simulink model "Custom_Inverter_Working_1 1"  (R2024a)
settings: Solver=FixedStepAuto  StartTime=0.0  StopTime=40  FixedStep=1e-5  MaxStep=1e-4  RelTol=1e-3
values from neighbouring files (symbols this model uses):
  A_f = 1.24    [Inverter_Working 1.m]
  C_d = 0.7041    [Inverter_Working 1.m]
  C_rr = 0.02    [Inverter_Working 1.m]
  g = 9.8    [Inverter_Working 1.m]
  J = mrot*r^2/k^2 + 0.0045    (= 0.8303048)    [Inverter_Working 1.m]
  k = 1    [Inverter_Working 1.m]
  lambda = 0.0375    [Inverter_Working 1.m]
  Ld = 0.1e-3    (= 0.0001)    [Inverter_Working 1.m]
  Lq = Ld    (= 0.0001)    [Inverter_Working 1.m]
  m = 371    [Inverter_Working 1.m]
  ppair = 1    [Inverter_Working 1.m]
  r = 0.4064/2    (= 0.2032)    [Inverter_Working 1.m]
  rho = 1.2    [Inverter_Working 1.m]
  Rs = 1.3e-3    (= 0.0013)    [Inverter_Working 1.m]
  V_bat = 24 * 3.6    (= 86.4)    [Inverter_Working 1.m]
undefined symbols (not defined in the file or in its folder): Down, Up
libraries: nesl_utility x12, fl_lib x6, ee_lib x5, slpidlib x3, simulink x2, spsabctodq0Lib x2, spsdq0toabcLib x2, eePwmGenerator x1
settings Model: Creator=cviana  LastModifiedBy=didad
settings RTWCC: GPUComputeCapability=3.5

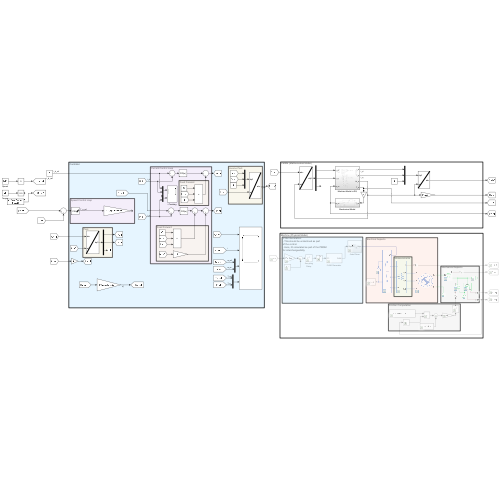
[thumbnail: Simulink's stored preview of the top-level diagram]
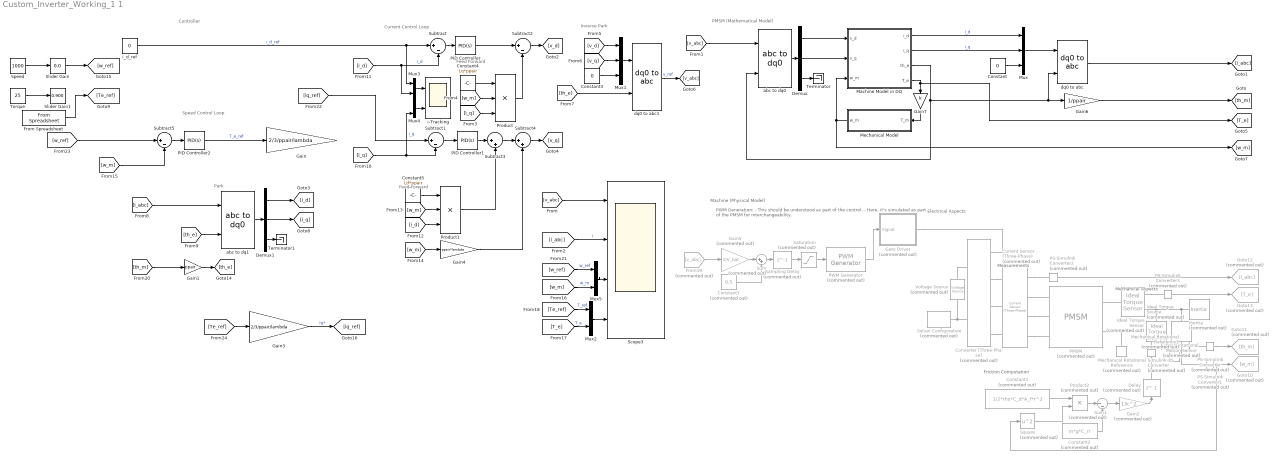
== system Custom_Inverter_Working_1 1 ==
  note: Friction Computation
  note: Machine (Physical Model)
  note: Feed Forward
  note: Feed Forward
  note: Current Control Loop
  note: Speed Control Loop
  note: Measurements
  note: Mechanical Aspects
  note: Electrical Aspects
  note: Park
  note: Inverse Park
  note: Controller
  note: PMSM (Mathematical Model)
  note: PWM Generation:
      | - This should be understood as part
      | of the control.
      | - Here, it's simulated as part of the PMSM
      | for interchangeability.
  Constant : Constant  Value=0
  Constant1 : Constant  Commented=on  Value=1/2*rho*C_d*A_f*r^2
  Constant2 : Constant  Commented=on  Value=m*g*C_rr
  Constant3 : Constant  Value=0
  Constant4 : Constant  Value=Lq*ppair
  Constant5 : Constant  Value=Ld*ppair
  Constant7 : Constant  Commented=on  Value=0.5
  Converter (Three-Phase) : ee_lib/Semiconductors & Converters/Converters/Converter (Three-Phase)  Commented=on  port_option=ee.enum.threePhasePort.expanded  fidelity_option=ee.enum.converters.fidelity.detailed  device_type=ee.enum.converters.switchingdevice.ideal  K=0  Vf=0.8 V  Ron=0.001 Ohm  Rds=0.001 Ohm  Goff=1e-6 1/Ohm  Vgt=1 V  Vgt_off=-1 V  Ih=1 A  Vth=6 V  diode_param=ee.enum.converters.protectiondiode.none  diode_Vf=0.8 V  diode_Ron=0.001 Ohm  diode_Goff=1e-5 1/Ohm  diode_C=50 nF  diode_iRM=-235 A  diode_iF=300 A  diode_idot=-50 A/us  diode_trr_param=ee.enum.converters.diodetrr.trr_factor  diode_trr_factor=3  diode_trr=15 us  diode_Qrr=1500 s*uA  snubber_type=ee.enum.converters.snubber.exclude  Cs=1e-7 F  Rs=0.1 Ohm
      settings: InternalSimscapePortConfiguration="{\"Bottom\":[],\"Left\":[{\"id\":\"G\",\"label\":\"G\",\"type\":\"foundation.electrical.twelve_phase\"},{\"id\":\"a\",\"label\":\"a\",\"type\":\"foundation.electrical.electrical\"},{\"id\":\"b\",\"label\":\"b\",\"type\":\"foundation.electrical.electrical\"},{\"id\":\"c\",\"label\":\"c\",\"type\":\"foundation.electrical.electrical\"}],\"Right\":[{\"id\":\"p\",\"label\":\"+\",\"type\":\"foundation.electrical.electrical\"},{\"id\":\"n\",\"label\":\"-\",\"type\":\"foundation.electrical.electrical\"}],\"Top\":[]}"
  Current Sensor (Three-Phase) : ee_lib/Sensors & Transducers/Current Sensor (Three-Phase)  Commented=on
      settings: InternalSimscapePortConfiguration="{\"Bottom\":[],\"Left\":[{\"id\":\"a1\",\"label\":\"a1\",\"type\":\"foundation.electrical.electrical\"},{\"id\":\"b1\",\"label\":\"b1\",\"type\":\"foundation.electrical.electrical\"},{\"id\":\"c1\",\"label\":\"c1\",\"type\":\"foundation.electrical.electrical\"}],\"Right\":[{\"id\":\"I_output\",\"label\":\"I\",\"type\":\"output\"},{\"id\":\"a2\",\"label\":\"a2\",\"type\":\"foundation.electrical.electrical\"},{\"id\":\"b2\",\"label\":\"b2\",\"type\":\"foundation.electrical.electrical\"},{\"id\":\"c2\",\"label\":\"c2\",\"type\":\"foundation.electrical.electrical\"}],\"Top\":[]}"
  Delay : Delay  Commented=on  DelayLength=1
  Demux : Demux  Outputs=3
  Demux1 : Demux  Outputs=3
  From Spreadsheet : FromSpreadsheet  FileName=Inverter_Lap_Sim_Current_Calcs.xlsx
  From19 : From  Commented=on  GotoTag=v_abc
  Gain : Gain  Gain=2/3/ppair/lambda
  Gain1 : Gain  Gain=ppair
  Gain2 : Gain  Commented=on  Gain=1/k^2
  Gain3 : Gain  Gain=2/3/ppair/lambda
  Gain4 : Gain  Gain=ppair*lambda
  Gain5 : Gain  Commented=on  Gain=1/V_bat
  Gain6 : Gain  Gain=1/ppair
  Gain7 : Gain  Gain=k
  Gate Driver : Subsystem  Commented=on
  Goto10 : Goto  Commented=on  GotoTag=w_m
  Goto11 : Goto  Commented=on  GotoTag=th_m
  Goto12 : Goto  Commented=on  GotoTag=i_abc
  Goto13 : Goto  Commented=on  GotoTag=T_e
  Ideal Rotational Motion Sensor : fl_lib/Mechanical/Mechanical Sensors/Ideal Rotational Motion Sensor  Commented=on  reference=foundation.enum.MeasurementReference.difference  acceleration_port=false  velocity_port=true  position_port=true  wrap_angle=false  offset=0 rad
  Ideal Torque Sensor : fl_lib/Mechanical/Mechanical Sensors/Ideal Torque Sensor  Commented=on
  Ideal Torque Source : fl_lib/Mechanical/Mechanical Sources/Ideal Torque Source  Commented=on
  Inertia : fl_lib/Mechanical/Rotational Elements/Inertia  Commented=on  inertia=J kg*m^2  num_ports=foundation.enum.numPorts2.one  w_specify=off  w_priority=High  w=0 rad/s  w_nominal_specify=off  w_nominal_value=1  w_nominal_unit=rad/s  t_specify=off  t_priority=None  t=0 N*m  t_nominal_specify=off  t_nominal_value=1  t_nominal_unit=N*m
  Machine Model in DQ : Subsystem
  Mechanical Rotational Reference : fl_lib/Mechanical/Rotational Elements/Mechanical Rotational Reference  Commented=on
  Mechanical Rotational Reference1 : fl_lib/Mechanical/Rotational Elements/Mechanical Rotational Reference  Commented=on
  Mechanical Model : Subsystem
  Mux : Mux  Inputs=3
  Mux1 : Mux  Inputs=3
  Mux{2..5} (4 alike) : Mux  Inputs=2
  PID Controller : slpidlib/PID Controller  Controller=PID  Form=Parallel  TimeDomain=Continuous-time  UseExternalTs=off  SampleTime=-1  IntegratorMethod=Forward Euler  FilterMethod=Forward Euler  ControllerParametersSource=internal  P=0.3  I=5  UseKiTs=off  D=0  UseExternalDerivativeSource=off  N=100  UseFilter=on  TunerSelectOption=Transfer Function Based (PID Tuner App)  InitialConditionSource=internal  InitialConditionForIntegrator=0  InitialConditionForFilter=0  DifferentiatorICPrevScaledInput=0  ExternalReset=none  TrackingMode=off  Kt=1  LimitOutput=off  SatLimitsSource=internal  UpperSaturationLimit=inf  LowerSaturationLimit=-inf  LinearizeAsGain=on  AntiWindupMode=none  Kb=1  LimitIntegrator=off  UpperIntegratorSaturationLimit=inf  LowerIntegratorSaturationLimit=-inf  POutMin=[]  POutMax=[]  IOutMin=[]  IOutMax=[]  DOutMin=[]  DOutMax=[]  NOutMin=[]  NOutMax=[]  SumOutMin=[]  SumOutMax=[]  SaturationOutMin=[]  SaturationOutMax=[]  PParamMin=[]  PParamMax=[]  IParamMin=[]  IParamMax=[]  DParamMin=[]  DParamMax=[]  NParamMin=[]  NParamMax=[]  KbParamMin=[]  KbParamMax=[]  KtParamMin=[]  KtParamMax=[]  KbOutMin=[]  KbOutMax=[]  KtOutMin=[]  KtOutMax=[]  IntegratorOutMin=[]  IntegratorOutMax=[]  FilterOutMin=[]  FilterOutMax=[]  SumI1OutMin=[]  SumI1OutMax=[]  SumI2OutMin=[]  SumI2OutMax=[]  SumI3OutMin=[]  SumI3OutMax=[]  SumI4OutMin=[]  SumI4OutMax=[]  SumDOutMin=[]  SumDOutMax=[]  DifferentiatorOutMin=[]  DifferentiatorOutMax=[]  FilterDiffOutCoefMin=[]  FilterDiffOutCoefMax=[]  ReciprocalOutMin=[]  ReciprocalOutMax=[]  SumDenOutMin=[]  SumDenOutMax=[]  SumNumOutMin=[]  SumNumOutMax=[]  DivideOutMin=[]  DivideOutMax=[]  UdiffTsProdOutMin=[]  UdiffTsProdOutMax=[]  NTsProdOutMin=[]  NTsProdOutMax=[]  UintegralTsProdOutMin=[]  UintegralTsProdOutMax=[]  UngainTsProdOutMin=[]  UngainTsProdOutMax=[]  ClampingZeroOutDataTypeStr=Inherit: Inherit via back propagation  ClampingZeroOutMin=[]  ClampingZeroOutMax=[]  FilterDenConstantOutDataTypeStr=Inherit: Inherit via back propagation  FilterDenConstantOutMin=[]  FilterDenConstantOutMax=[]  PCopyOutDataTypeStr=Inherit: Inherit via back propagation  PCopyOutMin=[]  PCopyOutMax=[]  NCopyOutDataTypeStr=Inherit: Inherit via back propagation  NCopyOutMin=[]  NCopyOutMax=[]  IntegratorContinuousStateAttributes=''  IntegratorStateMustResolveToSignalObject=off  IntegratorRTWStateStorageClass=Auto  FilterContinuousStateAttributes=''  FilterStateMustResolveToSignalObject=off  FilterRTWStateStorageClass=Auto  ParallelPVariant=InternalParameters  IdealPVariant=Disabled  IVariant=InternalParameters  DVariant=InternalParameters  IntegratorVariant=Continuous  SatVariant=Disabled  AWVariant=Passthrough  PCopyVariant=Disabled  TRVariant=Disabled  FdbkBlocksVariant=Forward  IdealPFdbkVariant=Disabled  SatFdbkVariant=Disabled  DerivativeFilterVariant=ContFilter  NVariant=InternalParameters  NCopyVariant=Disabled  FilterICVariant=InternalICsFilter  IntegratorICVariant=InternalICs  ExternalResetVariant=Disabled  TRSumVariant=Passthrough  SumFdbkVariant=Disabled  SumVariant=Sum_PID  TsampFilterVariant=InternalTs  TsampNgainVariant=Passthrough  TsampIntegralVariant=Disabled_SignalSpec  ExternalSaturationOutDataTypeStr=Inherit: Same as second input  DerivativeSourceVariant=ErrorSignal
  PID Controller1 : slpidlib/PID Controller  Controller=PID  Form=Parallel  TimeDomain=Continuous-time  UseExternalTs=off  SampleTime=-1  IntegratorMethod=Forward Euler  FilterMethod=Forward Euler  ControllerParametersSource=internal  P=0.3  I=5  UseKiTs=off  D=0  UseExternalDerivativeSource=off  N=100  UseFilter=on  TunerSelectOption=Transfer Function Based (PID Tuner App)  InitialConditionSource=internal  InitialConditionForIntegrator=0  InitialConditionForFilter=0  DifferentiatorICPrevScaledInput=0  ExternalReset=none  TrackingMode=off  Kt=1  LimitOutput=off  SatLimitsSource=internal  UpperSaturationLimit=inf  LowerSaturationLimit=-inf  LinearizeAsGain=on  AntiWindupMode=none  Kb=1  LimitIntegrator=off  UpperIntegratorSaturationLimit=inf  LowerIntegratorSaturationLimit=-inf  POutMin=[]  POutMax=[]  IOutMin=[]  IOutMax=[]  DOutMin=[]  DOutMax=[]  NOutMin=[]  NOutMax=[]  SumOutMin=[]  SumOutMax=[]  SaturationOutMin=[]  SaturationOutMax=[]  PParamMin=[]  PParamMax=[]  IParamMin=[]  IParamMax=[]  DParamMin=[]  DParamMax=[]  NParamMin=[]  NParamMax=[]  KbParamMin=[]  KbParamMax=[]  KtParamMin=[]  KtParamMax=[]  KbOutMin=[]  KbOutMax=[]  KtOutMin=[]  KtOutMax=[]  IntegratorOutMin=[]  IntegratorOutMax=[]  FilterOutMin=[]  FilterOutMax=[]  SumI1OutMin=[]  SumI1OutMax=[]  SumI2OutMin=[]  SumI2OutMax=[]  SumI3OutMin=[]  SumI3OutMax=[]  SumI4OutMin=[]  SumI4OutMax=[]  SumDOutMin=[]  SumDOutMax=[]  DifferentiatorOutMin=[]  DifferentiatorOutMax=[]  FilterDiffOutCoefMin=[]  FilterDiffOutCoefMax=[]  ReciprocalOutMin=[]  ReciprocalOutMax=[]  SumDenOutMin=[]  SumDenOutMax=[]  SumNumOutMin=[]  SumNumOutMax=[]  DivideOutMin=[]  DivideOutMax=[]  UdiffTsProdOutMin=[]  UdiffTsProdOutMax=[]  NTsProdOutMin=[]  NTsProdOutMax=[]  UintegralTsProdOutMin=[]  UintegralTsProdOutMax=[]  UngainTsProdOutMin=[]  UngainTsProdOutMax=[]  ClampingZeroOutDataTypeStr=Inherit: Inherit via back propagation  ClampingZeroOutMin=[]  ClampingZeroOutMax=[]  FilterDenConstantOutDataTypeStr=Inherit: Inherit via back propagation  FilterDenConstantOutMin=[]  FilterDenConstantOutMax=[]  PCopyOutDataTypeStr=Inherit: Inherit via back propagation  PCopyOutMin=[]  PCopyOutMax=[]  NCopyOutDataTypeStr=Inherit: Inherit via back propagation  NCopyOutMin=[]  NCopyOutMax=[]  IntegratorContinuousStateAttributes=''  IntegratorStateMustResolveToSignalObject=off  IntegratorRTWStateStorageClass=Auto  FilterContinuousStateAttributes=''  FilterStateMustResolveToSignalObject=off  FilterRTWStateStorageClass=Auto  ParallelPVariant=InternalParameters  IdealPVariant=Disabled  IVariant=InternalParameters  DVariant=InternalParameters  IntegratorVariant=Continuous  SatVariant=Disabled  AWVariant=Passthrough  PCopyVariant=Disabled  TRVariant=Disabled  FdbkBlocksVariant=Forward  IdealPFdbkVariant=Disabled  SatFdbkVariant=Disabled  DerivativeFilterVariant=ContFilter  NVariant=InternalParameters  NCopyVariant=Disabled  FilterICVariant=InternalICsFilter  IntegratorICVariant=InternalICs  ExternalResetVariant=Disabled  TRSumVariant=Passthrough  SumFdbkVariant=Disabled  SumVariant=Sum_PID  TsampFilterVariant=InternalTs  TsampNgainVariant=Passthrough  TsampIntegralVariant=Disabled_SignalSpec  ExternalSaturationOutDataTypeStr=Inherit: Same as second input  DerivativeSourceVariant=ErrorSignal
  PID Controller2 : slpidlib/PID Controller  Controller=PID  Form=Parallel  TimeDomain=Continuous-time  UseExternalTs=off  SampleTime=-1  IntegratorMethod=Forward Euler  FilterMethod=Forward Euler  ControllerParametersSource=internal  P=2.5  I=1.5  UseKiTs=off  D=0  UseExternalDerivativeSource=off  N=100  UseFilter=on  TunerSelectOption=Transfer Function Based (PID Tuner App)  InitialConditionSource=internal  InitialConditionForIntegrator=0  InitialConditionForFilter=0  DifferentiatorICPrevScaledInput=0  ExternalReset=none  TrackingMode=off  Kt=1  LimitOutput=on  SatLimitsSource=internal  UpperSaturationLimit=300  LowerSaturationLimit=-300  LinearizeAsGain=on  AntiWindupMode=back-calculation  Kb=1  LimitIntegrator=off  UpperIntegratorSaturationLimit=inf  LowerIntegratorSaturationLimit=-inf  POutMin=[]  POutMax=[]  IOutMin=[]  IOutMax=[]  DOutMin=[]  DOutMax=[]  NOutMin=[]  NOutMax=[]  SumOutMin=[]  SumOutMax=[]  SaturationOutMin=[]  SaturationOutMax=[]  PParamMin=[]  PParamMax=[]  IParamMin=[]  IParamMax=[]  DParamMin=[]  DParamMax=[]  NParamMin=[]  NParamMax=[]  KbParamMin=[]  KbParamMax=[]  KtParamMin=[]  KtParamMax=[]  KbOutMin=[]  KbOutMax=[]  KtOutMin=[]  KtOutMax=[]  IntegratorOutMin=[]  IntegratorOutMax=[]  FilterOutMin=[]  FilterOutMax=[]  SumI1OutMin=[]  SumI1OutMax=[]  SumI2OutMin=[]  SumI2OutMax=[]  SumI3OutMin=[]  SumI3OutMax=[]  SumI4OutMin=[]  SumI4OutMax=[]  SumDOutMin=[]  SumDOutMax=[]  DifferentiatorOutMin=[]  DifferentiatorOutMax=[]  FilterDiffOutCoefMin=[]  FilterDiffOutCoefMax=[]  ReciprocalOutMin=[]  ReciprocalOutMax=[]  SumDenOutMin=[]  SumDenOutMax=[]  SumNumOutMin=[]  SumNumOutMax=[]  DivideOutMin=[]  DivideOutMax=[]  UdiffTsProdOutMin=[]  UdiffTsProdOutMax=[]  NTsProdOutMin=[]  NTsProdOutMax=[]  UintegralTsProdOutMin=[]  UintegralTsProdOutMax=[]  UngainTsProdOutMin=[]  UngainTsProdOutMax=[]  ClampingZeroOutDataTypeStr=Inherit: Inherit via back propagation  ClampingZeroOutMin=[]  ClampingZeroOutMax=[]  FilterDenConstantOutDataTypeStr=Inherit: Inherit via back propagation  FilterDenConstantOutMin=[]  FilterDenConstantOutMax=[]  PCopyOutDataTypeStr=Inherit: Inherit via back propagation  PCopyOutMin=[]  PCopyOutMax=[]  NCopyOutDataTypeStr=Inherit: Inherit via back propagation  NCopyOutMin=[]  NCopyOutMax=[]  IntegratorContinuousStateAttributes=''  IntegratorStateMustResolveToSignalObject=off  IntegratorRTWStateStorageClass=Auto  FilterContinuousStateAttributes=''  FilterStateMustResolveToSignalObject=off  FilterRTWStateStorageClass=Auto  ParallelPVariant=InternalParameters  IdealPVariant=Disabled  IVariant=InternalParameters  DVariant=InternalParameters  IntegratorVariant=Continuous  SatVariant=Enabled  AWVariant=BackCalculation  PCopyVariant=Disabled  TRVariant=Disabled  FdbkBlocksVariant=Forward  IdealPFdbkVariant=Disabled  SatFdbkVariant=Disabled  DerivativeFilterVariant=ContFilter  NVariant=InternalParameters  NCopyVariant=Disabled  FilterICVariant=InternalICsFilter  IntegratorICVariant=InternalICs  ExternalResetVariant=Disabled  TRSumVariant=Passthrough  SumFdbkVariant=Disabled  SumVariant=Sum_PID  TsampFilterVariant=InternalTs  TsampNgainVariant=Passthrough  TsampIntegralVariant=Disabled_SignalSpec  ExternalSaturationOutDataTypeStr=Inherit: Same as second input  DerivativeSourceVariant=ErrorSignal
  PMSM : ee_lib/Electromechanical/Permanent Magnet/PMSM  Commented=on  port_option=ee.enum.threePhasePort.expanded  winding_type=ee.enum.statorconnection.wye  machine_param=ee.enum.pmsm.parameterization.constant  nPolePairs=p  pmflux_param=ee.enum.pmflux.fluxlinkage  pm_flux_linkage=lambda N*m/A  torque_constant=0.18 N*m/A  back_emf_constant=0.18 V*s/rad  stator_param=ee.enum.statorparam.LdLqL0  Ld=L_d H  Lq=L_q H  idVec=[-200, 0, 200] A  iqVec=[-200, 0, 200] A  LdMatrix=0.0002 * ones(3, 3) H  LqMatrix=0.0002 * ones(3, 3) H  PmMatrix=0.1 * ones(3, 3) Wb  ktMatrix=0.18 * ones(3, 3) N*m/A  keMatrix=0.18 * ones(3, 3) V*s/rad  L0=0.00016 H  Ls=0.0002 H  Lm=-0.00002 H  Ms=0.00002 H  Rs=R Ohm  zero_sequence=ee.enum.park.zerosequence.exclude  axes_param=ee.enum.rotorangle.daxis  loss_param=ee.enum.ironloss.none  losses_oc=[0, 0, 0] W  losses_sc=[0, 0, 0] W  f_losses=60 Hz  Isc_losses=95 A  J=0.000001 kg*m^2  lam=0 N*m*s/rad  i_d_specify=off  i_d_priority=None  i_d=0 A  i_d_nominal_specify=off  i_d_nominal_value=1  i_d_nominal_unit=A  i_q_specify=off  i_q_priority=None  i_q=0 A  i_q_nominal_specify=off  i_q_nominal_value=1  i_q_nominal_unit=A  torque_specify=off  torque_priority=None  torque=0 N*m  torque_nominal_specify=off  torque_nominal_value=1  torque_nominal_unit=N*m  angular_velocity_specify=off  angular_velocity_priority=High  angular_velocity=0 rpm  angular_velocity_nominal_specify=off  angular_velocity_nominal_value=1  angular_velocity_nominal_unit=rpm  angular_position_specify=off  angular_position_priority=High  angular_position=0 deg  angular_position_nominal_specify=off  angular_position_nominal_value=1  angular_position_nominal_unit=deg  alpha=3.93e-3 1/K  alpha_flux=-0.001 1/K  Tmeas=298.15 K  stator_thermal_mass=100 J/K  rotor_thermal_mass=200 J/K  Rm_percent_rotor=90  Rd_percent_rotor=30  temperatureA_specify=off  temperatureA_priority=High  temperatureA=25 degC  temperatureA_nominal_specify=off  temperatureA_nominal_value=1  temperatureA_nominal_unit=degC  temperatureB_specify=off  temperatureB_priority=High  temperatureB=25 degC  temperatureB_nominal_specify=off  temperatureB_nominal_value=1  temperatureB_nominal_unit=degC  temperatureC_specify=off  temperatureC_priority=High  temperatureC=25 degC  temperatureC_nominal_specify=off  temperatureC_nominal_value=1  temperatureC_nominal_unit=degC  temperatureR_specify=off  temperatureR_priority=High  temperatureR=25 degC  temperatureR_nominal_specify=off  temperatureR_nominal_value=1  temperatureR_nominal_unit=degC
      settings: InternalSimscapePortConfiguration="{\"Bottom\":[],\"Left\":[{\"id\":\"a\",\"label\":\"a\",\"type\":\"foundation.electrical.electrical\"},{\"id\":\"b\",\"label\":\"b\",\"type\":\"foundation.electrical.electrical\"},{\"id\":\"c\",\"label\":\"c\",\"type\":\"foundation.electrical.electrical\"}],\"Right\":[{\"id\":\"R\",\"label\":\"R\",\"type\":\"foundation.mechanical.rotational.rotational\"},{\"id\":\"C\",\"label\":\"C\",\"type\":\"foundation.mechanical.rotational.rotational\"}],\"Top\":[]}"
  PS-Simulink Converter{,1..3} (4 alike) : nesl_utility/PS-Simulink Converter  Commented=on  PhysicalDomain=network_engine_domain  SubClassName=ps_output  LeftPortType=input  RightPortType=output  PseudoPeriodic=off  Frequencies=[]  VectorFormat=inherit  Unit=inherit  AffineConversion=off
  PWM Generator : eePwmGenerator/PWM Generator  Commented=on  CarrCount=Up-Down  Tper=0.5/10e3  Tdelay=0  Ts=1e-6
  Product : Product  Inputs=3
  Product1 : Product  Inputs=3
  Product2 : Product  Commented=on
  Sampling Delay : Delay  Commented=on  DelayLength=1  SampleTime=1e-6
  Saturation : Saturate  Commented=on  UpperLimit=1  LowerLimit=0
  Scope3 : Scope  NumInputPorts=4
  Simulink-PS Converter : nesl_utility/Simulink-PS Converter  Commented=on  PhysicalDomain=network_engine_domain  SubClassName=ps_input  LeftPortType=input  RightPortType=output  PseudoPeriodic=off  Frequencies=[]  NoiseDistribution=none  NoiseParameters=[]  Unit=1  AffineConversion=off  FilteringAndDerivatives=provide  SimscapeFilterOrder=1  InputFilterTimeConstant=0.001  UdotUserProvided=0
  Slider Gain : simulink/Math Operations/Slider Gain  gain=0.0  low=0  high=5
  Slider Gain1 : simulink/Math Operations/Slider Gain  gain=0.900  low=0  high=5
  Solver Configuration : nesl_utility/Solver Configuration  Commented=on  PhysicalDomain=network_engine_domain  SubClassName=solver  LeftPortType=input  RightPortType=generic  Tones=[]  Harmonics=[]  SimulateNoise=off  Profile=off  UseLocalSampling=off  EnableSwitchedLinearOptims=on  FrequencyDomain=off  UseCCode=off  RelTol=0.001  AbsTol=0.001  MinStep=1e-09  ToWorkspace=off  RevertToSquareIcSolve=off  NumHomotopyIterations=100  PhasorMode=off  PhasorModeNumHarmonics=1  ConsistencySolver=NEWTON_XTOL_AFTER_FTOL  IndexReductionMethod=None  DoDC=off  ResidualTolerance=1e-09  ConsistencyTolSource=GLOBAL  ConsistencyAbsTol=0.001  ConsistencyRelTol=0.001  ConsistencyTolFactor=0.001  UseLocalSolver=on  LocalSolverChoice=NE_TRAPEZOIDAL_ADVANCER  ResolveIndetEquations=on  FunctionEvalNumThread=1  LocalSolverSampleTime=1e-6  DoFixedCost=on  MaxNonlinIter=3  MaxModeIter=2  ComputeImpulses=off  ImpulseIterations=2  LinearAlgebra=auto  LinearAlgebraNumThread=0  EquationFormulation=NE_TIME_EF  DelaysMemoryBudget=1024  AutomaticFiltering=on  FilteringTimeConstant=0.001  PartitionStorageMethod=AS_NEEDED  PartitionMemoryBudget=1024  PartitionMethod=ROBUST  MultibodyUseLocalSolver=off  MultibodyLocalSolverChoice=ODE1  MultibodyLocalSolverSampleTime=0.001
  Speed : Constant  Value=1000
  Square : Math  Commented=on  Operator=square
  Subtract{,1..2,5} (4 alike) : Sum  Inputs=|+-
  Subtract3 : Sum  Inputs=|++
  Subtract4 : Sum  Inputs=|++
  Sum : Sum  Commented=on  Inputs=|++
  Sum1 : Sum  Commented=on  Inputs=|--
  Terminator : Terminator
  Terminator1 : Terminator
  Torque : Constant  Value=25
  Voltage Source : ee_lib/Sources/Voltage Source  Commented=on  dc_voltage=V_bat V  ac_voltage=0 V  ac_shift=0 rad  ac_frequency=60 Hz  noise_mode=ee.enum.sources.noise.Disabled  PSD=0 V^2/Hz  sample_time=1e-3 s  repeatability=ee.enum.sources.repeatability.NotRepeatable  user_seed=0  auto_seed=3890346746  i_specify=off  i_priority=None  i=0 A  i_nominal_specify=off  i_nominal_value=1  i_nominal_unit=A  v_specify=off  v_priority=None  v=0 V  v_nominal_specify=off  v_nominal_value=1  v_nominal_unit=V
  abc to dq0 : spsabctodq0Lib/abc to dq0  Alignment=Aligned with phase A axis
  abc to dq1 : spsabctodq0Lib/abc to dq0  Alignment=Aligned with phase A axis
  dq0 to abc : spsdq0toabcLib/dq0 to abc  Alignment=Aligned with phase A axis
  dq0 to abc1 : spsdq0toabcLib/dq0 to abc  Alignment=Aligned with phase A axis
  i-Tracking : Scope  NumInputPorts=2
  i_d_ref : Constant  Value=0
  wires:
  Mechanical Model/1(w_m) -> [w_m], Machine Model in DQ/3(w_m)
  Machine Model in DQ/3(th_e) -> abc to dq0/2, dq0 to abc/2, Gain6/1
  [v_abc] -> abc to dq0/1
  abc to dq0/1 -> Demux/1
  Demux/3 -> Terminator/1
  Machine Model in DQ/1(i_d) -> Mux/1  "i_d"
  Machine Model in DQ/2(i_q) -> Mux/2  "i_q"
  Constant/1 -> Mux/3
  [i_abc] -> Scope3/2  "i"
  Mux/1 -> dq0 to abc/1
  dq0 to abc/1 -> [i_abc]
  i_d_ref/1 -> Mux3/1, Subtract/1  "i_d_ref"
  Subtract/1 -> PID Controller/1
  Subtract1/1 -> PID Controller1/1
  Demux/1 -> Machine Model in DQ/1(v_d)
  Demux/2 -> Machine Model in DQ/2(v_q)
  Mux1/1 -> dq0 to abc1/1
  Constant3/1 -> Mux1/3
  [v_d] -> Mux1/1
  [v_q] -> Mux1/2
  [th_e] -> abc to dq1/2
  [i_abc] -> abc to dq1/1
  abc to dq1/1 -> Demux1/1
  Demux1/3 -> Terminator1/1
  Constant4/1 -> Product/1
  [w_m] -> Product/2
  [i_q] -> Product/3
  Product/1 -> Subtract2/2
  PID Controller/1 -> Subtract2/1
  Subtract2/1 -> [v_d]
  Demux1/2 -> [i_q]
  [i_q] -> Mux4/2, Subtract1/2  "i_q"
  Demux1/1 -> [i_d]
  [i_d] -> Mux3/2, Subtract/2  "i_d"
  Product1/1 -> Subtract3/2
  [w_m] -> Gain4/1
  Constant5/1 -> Product1/1
  [w_m] -> Product1/2
  [i_d] -> Product1/3
  Subtract3/1 -> Subtract4/1
  PID Controller1/1 -> Subtract3/1
  Subtract4/1 -> [v_q]
  Gain4/1 -> Subtract4/2
  [w_m] -> Subtract5/2
  Subtract5/1 -> PID Controller2/1
  PID Controller2/1 -> Gain/1  "T_e_ref"
  [Te_ref] -> Mux2/1  "T_ref"
  [T_e] -> Mux2/2  "T_e"
  Mux2/1 -> Scope3/4
  PS-Simulink Converter3/1 -> Goto13/1
  Gain1/1 -> [th_e]
  [th_m] -> Gain1/1
  Gain5/1 -> Sum/1
  Constant7/1 -> Sum/2
  PS-Simulink Converter2/1 -> Goto12/1
  PS-Simulink Converter/1 -> Goto11/1
  Sum/1 -> Sampling Delay/1
  [th_e] -> dq0 to abc1/2
  dq0 to abc1/1 -> [v_abc]  "v_ref"
  From19/1 -> Gain5/1
  Gain6/1 -> [th_m]
  Mux4/1 -> i-Tracking/2
  Mux3/1 -> i-Tracking/1
  [w_ref] -> Mux5/1  "w_ref"
  [w_m] -> Mux5/2  "w_m"
  Mux5/1 -> Scope3/3
  Sampling Delay/1 -> Saturation/1
  Saturation/1 -> PWM Generator/1
  [v_abc] -> Scope3/1
  PWM Generator/1 -> Gate Driver/1(Signal)
  Constant1/1 -> Product2/1
  PS-Simulink Converter1/1 -> Goto10/1, Square/1
  Square/1 -> Product2/2
  Product2/1 -> Sum1/1
  Constant2/1 -> Sum1/2
  Sum1/1 -> Gain2/1
  Gain2/1 -> Delay/1
  Delay/1 -> Simulink-PS Converter/1
  [w_ref] -> Subtract5/1
  Speed/1 -> Slider Gain/1
  Slider Gain/1 -> [w_ref]
  Gain3/1 -> [iq_ref]  "Iq*"
  [Te_ref] -> Gain3/1
  Torque/1 -> Slider Gain1/1
  [iq_ref] -> Subtract1/1
  Machine Model in DQ/4(T_e) -> [T_e], Gain7/1
  Gain7/1 -> Mechanical Model/1(T_m)
  From Spreadsheet/1 -> [Te_ref]
  connections:
  Ideal Rotational Motion Sensor/RConn3 -- PS-Simulink Converter/LConn1
  PS-Simulink Converter1/LConn1 -- Ideal Rotational Motion Sensor/RConn2
  PMSM/LConn1 -- Current Sensor (Three-Phase)/RConn2
  Current Sensor (Three-Phase)/RConn1 -- PS-Simulink Converter2/LConn1
  Current Sensor (Three-Phase)/RConn3 -- PMSM/LConn2
  Current Sensor (Three-Phase)/RConn4 -- PMSM/LConn3
  Ideal Torque Sensor/LConn1 -- PMSM/RConn1
  Ideal Torque Sensor/RConn2 -- PS-Simulink Converter3/LConn1
  Converter (Three-Phase)/LConn2 -- Current Sensor (Three-Phase)/LConn1
  Solver Configuration/RConn1 -- Voltage Source/RConn1 -- Converter (Three-Phase)/RConn2
  Converter (Three-Phase)/LConn3 -- Current Sensor (Three-Phase)/LConn2
  Converter (Three-Phase)/LConn4 -- Current Sensor (Three-Phase)/LConn3
  Voltage Source/LConn1 -- Converter (Three-Phase)/RConn1
  PMSM/RConn2 -- Mechanical Rotational Reference/LConn1
  Mechanical Rotational Reference1/LConn1 -- Ideal Torque Source/RConn2 -- Ideal Rotational Motion Sensor/RConn1
  Ideal Rotational Motion Sensor/LConn1 -- Inertia/LConn1 -- Ideal Torque Source/LConn1 -- Ideal Torque Sensor/RConn1
  Gate Driver/RConn1 -- Converter (Three-Phase)/LConn1
  Simulink-PS Converter/RConn1 -- Ideal Torque Source/RConn1

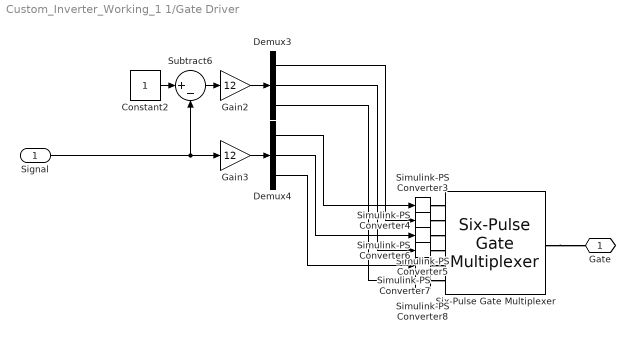
== system Custom_Inverter_Working_1 1/Gate Driver ==
  Signal : Inport
  Constant2 : Constant
  Demux3 : Demux  Outputs=3
  Demux4 : Demux  Outputs=3
  Gain2 : Gain  Gain=12
  Gain3 : Gain  Gain=12
  Simulink-PS Converter{3..8} (6 alike) : nesl_utility/Simulink-PS Converter  PhysicalDomain=network_engine_domain  SubClassName=ps_input  LeftPortType=input  RightPortType=output  PseudoPeriodic=off  Frequencies=[]  NoiseDistribution=none  NoiseParameters=[]  Unit=1  AffineConversion=off  FilteringAndDerivatives=provide  SimscapeFilterOrder=1  InputFilterTimeConstant=0.001  UdotUserProvided=0
  Six-Pulse Gate Multiplexer : ee_lib/Semiconductors & Converters/Converters/Six-Pulse Gate Multiplexer  port_option=ee.enum.controlport.ps
  Subtract6 : Sum  Inputs=|+-
  Gate : PMIOPort  Side=Right
  wires:
  Subtract6/1 -> Gain2/1
  Demux3/2 -> Simulink-PS Converter6/1
  Demux4/1 -> Simulink-PS Converter3/1
  Gain3/1 -> Demux4/1
  Demux3/3 -> Simulink-PS Converter8/1
  Demux4/3 -> Simulink-PS Converter7/1
  Signal/1 -> Gain3/1, Subtract6/2
  Demux4/2 -> Simulink-PS Converter5/1
  Gain2/1 -> Demux3/1
  Constant2/1 -> Subtract6/1
  Demux3/1 -> Simulink-PS Converter4/1
  connections:
  Simulink-PS Converter8/RConn1 -- Six-Pulse Gate Multiplexer/LConn6
  Simulink-PS Converter4/RConn1 -- Six-Pulse Gate Multiplexer/LConn2
  Simulink-PS Converter7/RConn1 -- Six-Pulse Gate Multiplexer/LConn5
  Simulink-PS Converter5/RConn1 -- Six-Pulse Gate Multiplexer/LConn3
  Simulink-PS Converter3/RConn1 -- Six-Pulse Gate Multiplexer/LConn1
  Simulink-PS Converter6/RConn1 -- Six-Pulse Gate Multiplexer/LConn4
  Six-Pulse Gate Multiplexer/RConn1 -- Gate/RConn1

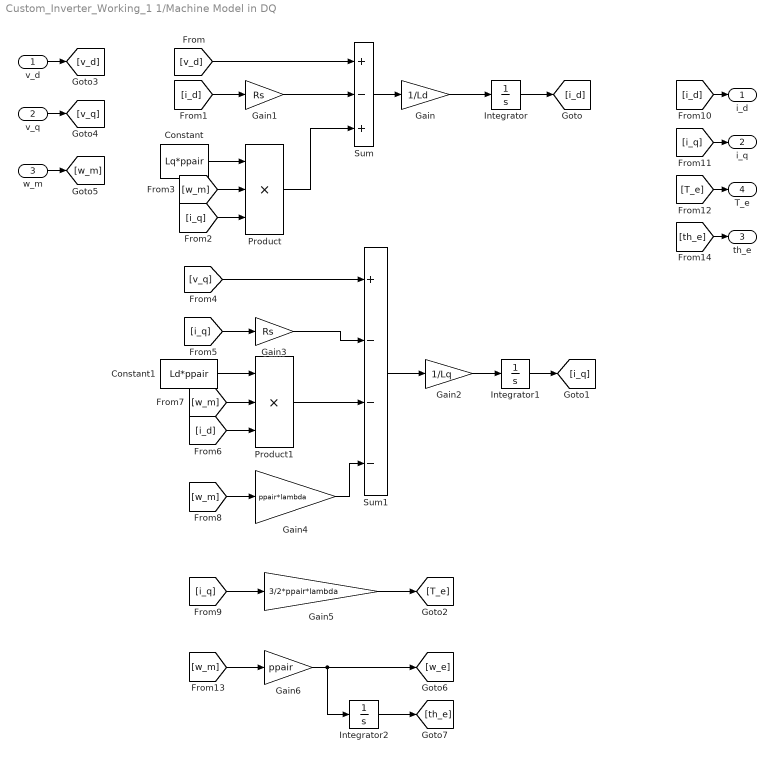
== system Custom_Inverter_Working_1 1/Machine Model in DQ ==
  v_d : Inport
  v_q : Inport  Port=2
  w_m : Inport  Port=3
  Constant : Constant  Value=Lq*ppair
  Constant1 : Constant  Value=Ld*ppair
  Gain : Gain  Gain=1/Ld
  Gain1 : Gain  Gain=Rs
  Gain2 : Gain  Gain=1/Lq
  Gain3 : Gain  Gain=Rs
  Gain4 : Gain  Gain=ppair*lambda
  Gain5 : Gain  Gain=3/2*ppair*lambda
  Gain6 : Gain  Gain=ppair
  Integrator : Integrator
  Integrator1 : Integrator
  Integrator2 : Integrator
  Product : Product  Inputs=3
  Product1 : Product  Inputs=3
  Sum : Sum  Inputs=+-+
  Sum1 : Sum  Inputs=+---
  i_d : Outport
  i_q : Outport  Port=2
  th_e : Outport  Port=3
  T_e : Outport  Port=4
  wires:
  Constant/1 -> Product/1
  Product/1 -> Sum/3
  Integrator/1 -> [i_d]
  [v_d] -> Sum/1
  [w_m] -> Product1/2
  Gain4/1 -> Sum1/4
  [i_q] -> Product/3
  Sum/1 -> Gain/1
  [w_m] -> Gain4/1
  [i_d] -> Gain1/1
  Sum1/1 -> Gain2/1
  Gain/1 -> Integrator/1
  Gain5/1 -> [T_e]
  [i_q] -> Gain5/1
  Gain1/1 -> Sum/2
  Integrator1/1 -> [i_q]
  [i_q] -> Gain3/1
  Product1/1 -> Sum1/3
  Constant1/1 -> Product1/1
  Gain2/1 -> Integrator1/1
  [v_q] -> Sum1/1
  Gain3/1 -> Sum1/2
  [i_d] -> Product1/3
  [w_m] -> Product/2
  v_d/1 -> [v_d]
  v_q/1 -> [v_q]
  [i_d] -> i_d/1
  [i_q] -> i_q/1
  [T_e] -> T_e/1
  w_m/1 -> [w_m]
  [w_m] -> Gain6/1
  Gain6/1 -> Integrator2/1, [w_e]
  Integrator2/1 -> [th_e]
  [th_e] -> th_e/1

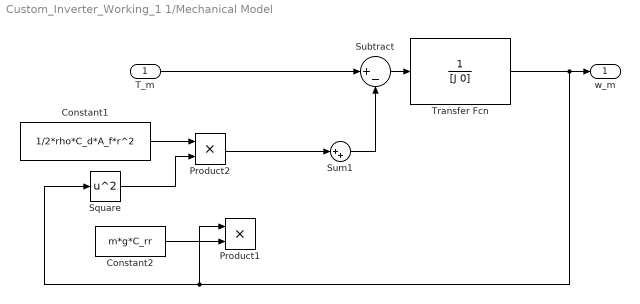
== system Custom_Inverter_Working_1 1/Mechanical Model ==
  T_m : Inport
  Constant1 : Constant  Value=1/2*rho*C_d*A_f*r^2
  Constant2 : Constant  Value=m*g*C_rr
  Product1 : Product
  Product2 : Product
  Square : Math  Operator=square
  Subtract : Sum  Inputs=|+-
  Sum1 : Sum  Inputs=|++
  Transfer Fcn : TransferFcn  Denominator=[J 0]
  w_m : Outport
  wires:
  Constant1/1 -> Product2/1
  Transfer Fcn/1 -> Product1/1, Square/1, w_m/1
  Square/1 -> Product2/2
  Subtract/1 -> Transfer Fcn/1
  Sum1/1 -> Subtract/2
  Product2/1 -> Sum1/1
  Constant2/1 -> Product1/2
  T_m/1 -> Subtract/1
